simulink library "setpointToOutput_cl"  (R2018b)
settings: Solver=VariableStepAuto  StartTime=0.0  StopTime=10.0  RelTol=1e-3
undefined symbols (not defined in the file): pathCtrl
libraries: filteredPIDController_ul x3, dynamicPressure_ul x1, eulAng2RotMat_ul x1, angleBtw2Vecs_ul x1, alphaBeta_ul x1, schmehlTangentRotation_ul x1
settings Model: Creator=jldanie5  LastModifiedBy=jldanie5

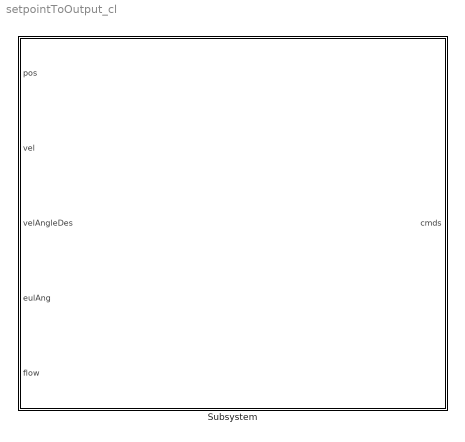
== system setpointToOutput_cl ==
  Subsystem : Subsystem

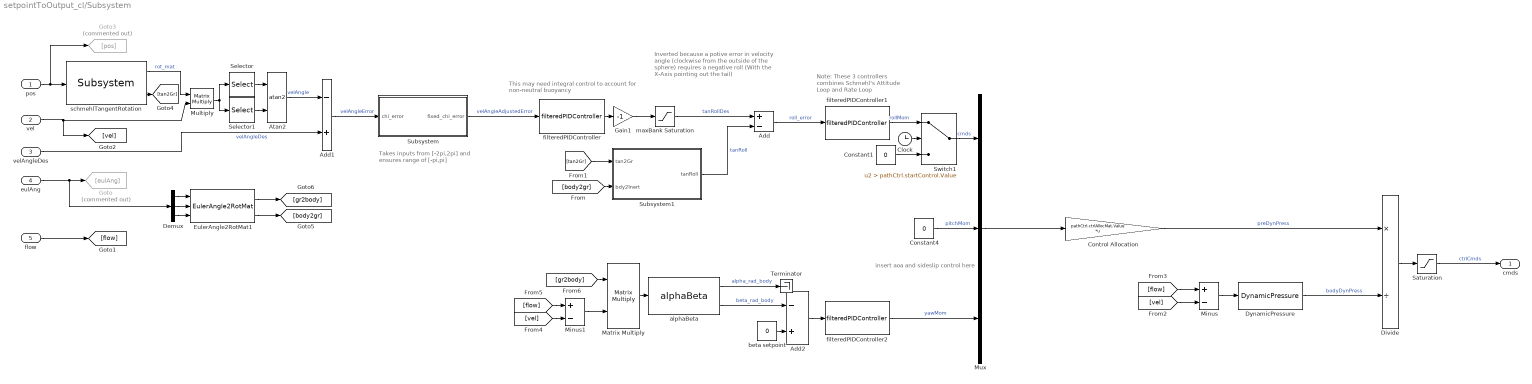
== system setpointToOutput_cl/Subsystem ==
  note: insert aoa and sideslip control here
  note: Inverted because a potive error
      | in velocity angle (clockwise from the
      | outside of the sphere) requires a negative
      | roll (With the X-Axis pointing out the tail)
  note: Note: These 3 controllers
      | combines Schmehl's Attitude
      | Loop and Rate Loop
  note: This may need integral control to account for
      | non-neutral buoyancy
  note: Takes inputs from [-2pi,2pi] and
      | ensures range of [-pi,pi]
  pos : Inport
  vel : Inport  Port=2
  velAngleDes : Inport  Port=3
  eulAng : Inport  Port=4
  flow : Inport  Port=5
  Add : Sum  Inputs=+-
  Add1 : Sum  Inputs=-+
  Add2 : Sum  Inputs=-+
  Atan2 : Trigonometry  Operator=atan2
  Clock : Clock
  Constant1 : Constant  Value=0
  Constant4 : Constant  Value=0
  Control Allocation : Gain  Gain=pathCtrl.ctrlAllocMat.Value  Multiplication=Matrix(K*u)
  Demux : Demux  Outputs=3
  Divide : Product  Inputs=*/
  DynamicPressure : dynamicPressure_ul/DynamicPressure  rho=fluidDensity
  EulerAngle2RotMat1 : eulAng2RotMat_ul/EulerAngle2RotMat  SystemSampleTime=-1
  Gain1 : Gain  Gain=-1
  Goto : Goto  Commented=on  GotoTag=eulAng
  Goto3 : Goto  Commented=on  GotoTag=pos
  Matrix Multiply : Product  Multiplication=Matrix(*)
  Minus : Sum  Inputs=+-
  Minus1 : Sum  Inputs=+-
  Multiply : Product  Multiplication=Matrix(*)
  Mux : Mux  Inputs=3
  Saturation : Saturate  UpperLimit=pathCtrl.controlSigMax.upperLimit.Value  LowerLimit=pathCtrl.controlSigMax.lowerLimit.Value
  Selector : Selector  InputPortWidth=3  IndexOptions=Index vector (dialog)  Indices=2  OutputSizes=1
  Selector1 : Selector  InputPortWidth=3  IndexOptions=Index vector (dialog)  Indices=1  OutputSizes=1
  Subsystem : Subsystem
  Subsystem1 : Subsystem
  Switch1 : Switch  Criteria=u2 > Threshold  Threshold=pathCtrl.startControl.Value
  Terminator : Terminator
  alphaBeta : alphaBeta_ul/alphaBeta  SystemSampleTime=-1
  beta setpoint : Constant  Value=0
  filteredPIDController : filteredPIDController_ul/filteredPIDController  kp=pathCtrl.velAng.kp.Value  ki=0  kd=pathCtrl.velAng.kd.Value  Value=pathCtrl.velAng.tau.Value
  filteredPIDController1 : filteredPIDController_ul/filteredPIDController  kp=pathCtrl.rollMoment.kp.Value  ki=0  kd=pathCtrl.rollMoment.kd.Value  Value=pathCtrl.rollMoment.tau.Value
  filteredPIDController2 : filteredPIDController_ul/filteredPIDController  kp=pathCtrl.yawMoment.kp.Value  ki=0  kd=pathCtrl.yawMoment.kd.Value  Value=pathCtrl.yawMoment.tau.Value
  maxBank Saturation : Saturate  UpperLimit=pathCtrl.maxBank.upperLimit.Value  LowerLimit=pathCtrl.maxBank.lowerLimit.Value
  schmehlTangentRotation : schmehlTangentRotation_ul/Subsystem  SystemSampleTime=-1
  cmds : Outport
  wires:
  schmehlTangentRotation/2 -> [tan2Gr]
  schmehlTangentRotation/1 -> Multiply/1  "rot_mat"
  pos/1 -> Goto3/1, schmehlTangentRotation/1
  vel/1 -> [vel], Multiply/2
  Multiply/1 -> Selector/1, Selector1/1
  Selector1/1 -> Atan2/2
  Selector/1 -> Atan2/1
  Atan2/1 -> Add1/1  "velAngle"
  velAngleDes/1 -> Add1/2  "velAngleDes"
  Add/1 -> filteredPIDController1/1  "roll_error"
  Subsystem/1(fixed_chi_error) -> filteredPIDController/1  "velAngleAdjustedError"
  filteredPIDController/1 -> Gain1/1
  Gain1/1 -> maxBank Saturation/1
  maxBank Saturation/1 -> Add/1  "tanRollDes"
  Add1/1 -> Subsystem/1(chi_error)  "velAngleError"
  Constant4/1 -> Mux/2  "pitchMom"
  flow/1 -> [flow]
  [tan2Gr] -> Subsystem1/1(tan2Gr)
  Subsystem1/1(tanRoll) -> Add/2  "tanRoll"
  Mux/1 -> Control Allocation/1
  [flow] -> Minus/1
  [vel] -> Minus/2
  Minus/1 -> DynamicPressure/1
  Control Allocation/1 -> Divide/1  "preDynPress"
  Divide/1 -> Saturation/1
  DynamicPressure/1 -> Divide/2  "bodyDynPress"
  Constant1/1 -> Switch1/3
  Clock/1 -> Switch1/2
  filteredPIDController1/1 -> Switch1/1  "rollMom"
  Switch1/1 -> Mux/1  "cmds"
  filteredPIDController2/1 -> Mux/3  "yawMom"
  Saturation/1 -> cmds/1  "ctrlCmds"
  Minus1/1 -> Matrix Multiply/2
  [vel] -> Minus1/2
  [flow] -> Minus1/1
  eulAng/1 -> Demux/1, Goto/1
  Demux/3 -> EulerAngle2RotMat1/3
  Demux/1 -> EulerAngle2RotMat1/1
  Demux/2 -> EulerAngle2RotMat1/2
  EulerAngle2RotMat1/2 -> [body2gr]
  EulerAngle2RotMat1/1 -> [gr2body]
  [body2gr] -> Subsystem1/2(bdy2Inert)
  [gr2body] -> Matrix Multiply/1
  Matrix Multiply/1 -> alphaBeta/1
  alphaBeta/1 -> Terminator/1  "alpha_rad_body"
  alphaBeta/2 -> Add2/1  "beta_rad_body"
  Add2/1 -> filteredPIDController2/1
  beta setpoint/1 -> Add2/2

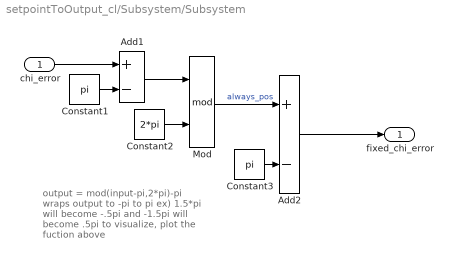
== system setpointToOutput_cl/Subsystem/Subsystem ==
  note: output = mod(input-pi,2*pi)-pi
      | wraps output to -pi to pi
      |
      | ex) 1.5*pi will become -.5pi
      | 	and -1.5pi will become .5pi
      |
      | to visualize, plot the fuction above
  chi_error : Inport
  Add1 : Sum  Inputs=+-
  Add2 : Sum  Inputs=+-
  Constant1 : Constant  Value=pi
  Constant2 : Constant  Value=2*pi
  Constant3 : Constant  Value=pi
  Mod : Math  Operator=mod  SaturateOnIntegerOverflow=on
  fixed_chi_error : Outport
  wires:
  chi_error/1 -> Add1/1
  Constant1/1 -> Add1/2
  Add1/1 -> Mod/1
  Constant2/1 -> Mod/2
  Mod/1 -> Add2/1  "always_pos"
  Constant3/1 -> Add2/2
  Add2/1 -> fixed_chi_error/1

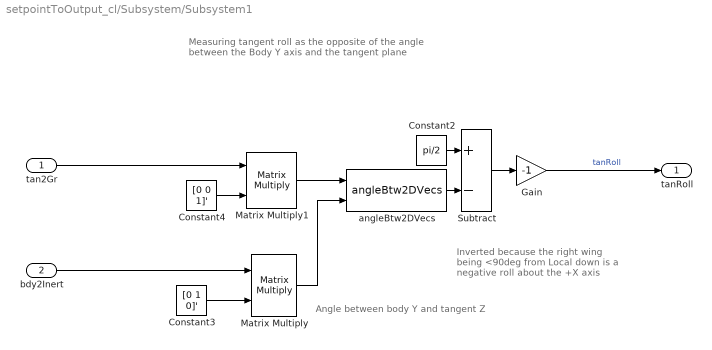
== system setpointToOutput_cl/Subsystem/Subsystem1 ==
  note: Measuring tangent roll as the opposite
      | of the angle between the Body Y axis
      | and the tangent plane
  note: Angle between body Y and tangent Z
  note: Inverted because the right wing
      | being <90deg from Local down
      | is a negative roll about the +X axis
  tan2Gr : Inport
  bdy2Inert : Inport  Port=2
  Constant2 : Constant  Value=pi/2
  Constant3 : Constant  Value=[0 1 0]'
  Constant4 : Constant  Value=[0 0 1]'
  Gain : Gain  Gain=-1
  Matrix Multiply : Product  Multiplication=Matrix(*)
  Matrix Multiply1 : Product  Multiplication=Matrix(*)
  Subtract : Sum  Inputs=+-
  angleBtw2DVecs : angleBtw2Vecs_ul/angleBtw2DVecs  SystemSampleTime=-1
  tanRoll : Outport
  wires:
  Constant3/1 -> Matrix Multiply/2
  angleBtw2DVecs/1 -> Subtract/2
  Constant2/1 -> Subtract/1
  Matrix Multiply1/1 -> angleBtw2DVecs/1
  Constant4/1 -> Matrix Multiply1/2
  Matrix Multiply/1 -> angleBtw2DVecs/2
  Subtract/1 -> Gain/1
  tan2Gr/1 -> Matrix Multiply1/1
  Gain/1 -> tanRoll/1  "tanRoll"
  bdy2Inert/1 -> Matrix Multiply/1
